simulink subsystem "Controllers"  (R2021b)
settings: Solver=VariableStepAuto  StartTime=0.0  StopTime=10.0  RelTol=1e-3
model mask{SurgeInitial=eta_IC.N, SurgeL=1.17*2, SurgeEpsilon=0.05, SurgeC0=3, SurgeAlpha=0.5, SwayInitial=eta_IC.E, SwayL=1.04, SwayEpsilon=0.03, SwayC0=3, SwayAlpha=0.5, HeaveInitial=eta_IC.D, HeaveL=0.7*5, HeaveEpsilon=0.05, HeaveC0=2, HeaveAlpha=0.1, RollInitial=eta_IC.phi, RollL=2.01, RollEpsilon=0.1, RollC0=0.4, RollAlpha=0.1, PitchInitial=eta_IC.theta, PitchL=1.83, PitchEpsilon=0.1, PitchC0=0.4, PitchAlpha=0.1, YawInitial=eta_IC.psi, YawL=2.05, YawEpsilon=0.1, YawC0=2, YawAlpha=0.1}
  mask prompts: SurgeInitial "Initial Condition"; SurgeL "L"; SurgeEpsilon "Epsilon"; SurgeC0 "C0"; SurgeAlpha "Alpha"; SwayInitial "Initial Condition"; SwayL "L"; SwayEpsilon "Epsilon"; SwayC0 "C0"; SwayAlpha "Alpha"; HeaveInitial "Initial Condition"; HeaveL "L"; HeaveEpsilon "Epsilon"; HeaveC0 "C0"; HeaveAlpha "Alpha"; RollInitial "Initial Condition"; RollL "L"; RollEpsilon "Epsilon"; RollC0 "C0"; RollAlpha "Alpha"; PitchInitial "Initial Condition"; PitchL "L"; PitchEpsilon "Epsilon"; PitchC0 "C0"; PitchAlpha "Alpha"; YawInitial "Initial Condition"; YawL "L"; YawEpsilon "Epsilon"; YawC0 "C0"; YawAlpha "Alpha"
undefined symbols (not defined in the file): eta_Init
libraries: simulink x12
settings Model: Creator=esben  LastModifiedBy=esben
settings SolverCC: AlgebraicLoopSolver=TrustRegion

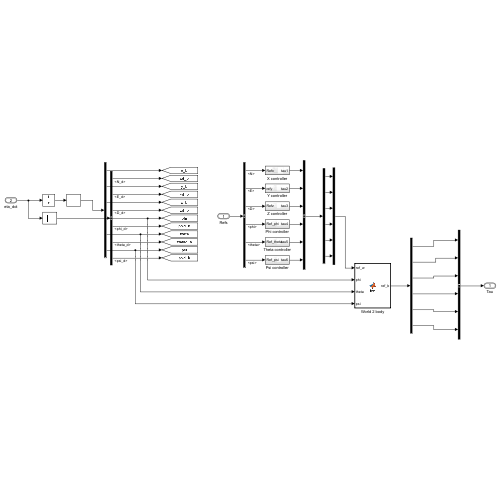
[thumbnail: Simulink's stored preview of the top-level diagram]
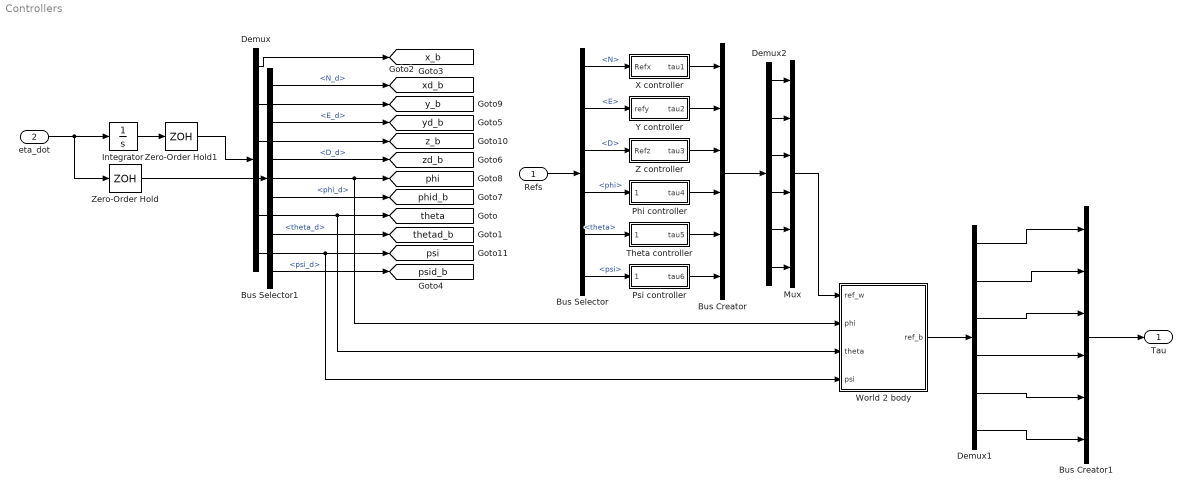
== system Controllers ==
  Refs : Inport  OutDataTypeStr=Bus: eta
  eta_dot : Inport  Port=2  OutDataTypeStr=Bus: nu
  Bus Creator : BusCreator  Inputs=6  OutDataTypeStr=Bus: tau
      settings: InheritFromInputs=off
  Bus Creator1 : BusCreator  Inputs=6  OutDataTypeStr=Bus: tau
      settings: InheritFromInputs=off
  Bus Selector : BusSelector  OutputSignals=N,E,D,phi,theta,psi
  Bus Selector1 : BusSelector  OutputSignals=N_d,E_d,D_d,phi_d,theta_d,psi_d
  Demux : Demux  Outputs=6
  Demux1 : Demux  Outputs=6
  Demux2 : Demux  Outputs=6
  Integrator : Integrator  InitialCondition=eta_Init
  Mux : Mux  Inputs=6
  Phi controller : Subsystem
  Psi controller : Subsystem
  Theta controller : Subsystem
  World 2 body : MATLAB Function  TreatAsAtomicUnit=on
  X controller : Subsystem
  Y controller : Subsystem
  Z controller : Subsystem
  Zero-Order Hold : ZeroOrderHold  SampleTime=1/20
  Zero-Order Hold1 : ZeroOrderHold  SampleTime=1/20
  Tau : Outport  OutDataTypeStr=Bus: tau
  tag scope: phi=global, phid_b=global, psi=global, psid_b=global, theta=global, thetad_b=global, x_b=global, xd_b=global, y_b=global, yd_b=global, z_b=global, zd_b=global
  wires:
  Theta controller/1(tau5) -> Bus Creator/5
  Bus Selector/5 -> Theta controller/1(Ref_theta)  "<theta>"
  Bus Selector/2 -> Y controller/1("refy ")  "<E>"
  Phi controller/1(tau4) -> Bus Creator/4
  Bus Selector/6 -> Psi controller/1(Ref_psi)  "<psi>"
  Psi controller/1(tau6) -> Bus Creator/6
  Z controller/1(tau3) -> Bus Creator/3
  Bus Selector/1 -> X controller/1(Refx)  "<N>"
  Bus Selector/4 -> Phi controller/1(Ref_phi)  "<phi>"
  Refs/1 -> Bus Selector/1
  Bus Selector/3 -> Z controller/1(Refz)  "<D>"
  eta_dot/1 -> Integrator/1, Zero-Order Hold/1
  Demux/5 -> [theta], World 2 body/3(theta)
  Bus Selector1/5 -> [thetad_b]  "<theta_d>"
  Bus Selector1/6 -> [psid_b]  "<psi_d>"
  Demux/1 -> [x_b]
  Bus Selector1/1 -> [xd_b]  "<N_d>"
  Bus Selector1/2 -> [yd_b]  "<E_d>"
  Bus Selector1/3 -> [zd_b]  "<D_d>"
  Demux/2 -> [y_b]
  Demux/3 -> [z_b]
  Demux/4 -> [phi], World 2 body/2(phi)
  Bus Selector1/4 -> [phid_b]  "<phi_d>"
  Demux/6 -> [psi], World 2 body/4(psi)
  Y controller/1(tau2) -> Bus Creator/2
  X controller/1(tau1) -> Bus Creator/1
  Zero-Order Hold/1 -> Bus Selector1/1
  Integrator/1 -> Zero-Order Hold1/1
  Zero-Order Hold1/1 -> Demux/1
  World 2 body/1(ref_b) -> Demux1/1
  Demux1/1 -> Bus Creator1/1
  Demux1/2 -> Bus Creator1/2
  Demux1/3 -> Bus Creator1/3
  Demux1/4 -> Bus Creator1/4
  Demux1/5 -> Bus Creator1/5
  Demux1/6 -> Bus Creator1/6
  Bus Creator1/1 -> Tau/1
  Bus Creator/1 -> Demux2/1
  Demux2/6 -> Mux/6
  Demux2/1 -> Mux/1
  Demux2/2 -> Mux/2
  Demux2/3 -> Mux/3
  Demux2/4 -> Mux/4
  Demux2/5 -> Mux/5
  Mux/1 -> World 2 body/1(ref_w)

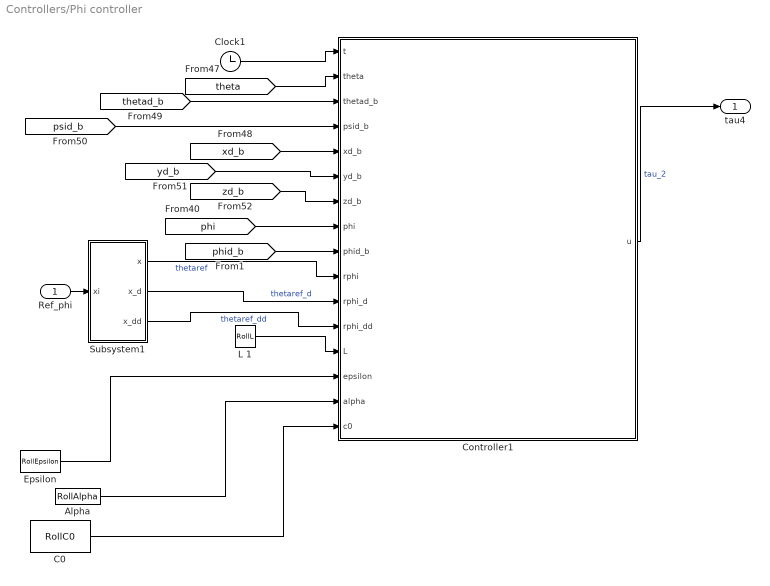
== system Controllers/Phi controller ==
  Ref_phi : Inport
  Alpha : Constant  Value=RollAlpha
  C0 : Constant  Value=RollC0
  Clock1 : Clock
  Controller1 : MATLAB Function  TreatAsAtomicUnit=on
  Epsilon : Constant  Value=RollEpsilon
  L 1 : Constant  Value=RollL
  Subsystem1 : Subsystem
  tau4 : Outport
  wires:
  C0/1 -> Controller1/16(c0)
  Epsilon/1 -> Controller1/14(epsilon)
  Alpha/1 -> Controller1/15(alpha)
  [phid_b] -> Controller1/9(phid_b)
  Controller1/1(u) -> tau4/1  "tau_2"
  Ref_phi/1 -> Subsystem1/1(xi)
  [xd_b] -> Controller1/5(xd_b)
  [psid_b] -> Controller1/4(psid_b)
  [zd_b] -> Controller1/7(zd_b)
  Subsystem1/1(x) -> Controller1/10(rphi)  "thetaref"
  [yd_b] -> Controller1/6(yd_b)
  Subsystem1/2(x_d) -> Controller1/11(rphi_d)  "thetaref_d"
  [phi] -> Controller1/8(phi)
  Clock1/1 -> Controller1/1(t)
  [thetad_b] -> Controller1/3(thetad_b)
  L 1/1 -> Controller1/13(L)
  [theta] -> Controller1/2(theta)
  Subsystem1/3(x_dd) -> Controller1/12(rphi_dd)  "thetaref_dd"

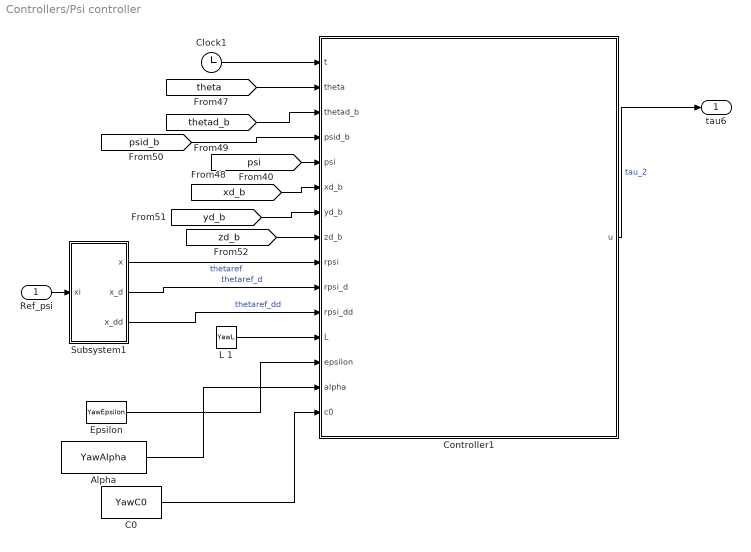
== system Controllers/Psi controller ==
  Ref_psi : Inport
  Alpha : Constant  Value=YawAlpha
  C0 : Constant  Value=YawC0
  Clock1 : Clock
  Controller1 : MATLAB Function  TreatAsAtomicUnit=on
  Epsilon : Constant  Value=YawEpsilon
  L 1 : Constant  Value=YawL
  Subsystem1 : Subsystem
  tau6 : Outport
  wires:
  Controller1/1(u) -> tau6/1  "tau_2"
  Ref_psi/1 -> Subsystem1/1(xi)
  C0/1 -> Controller1/15(c0)
  [xd_b] -> Controller1/6(xd_b)
  [psid_b] -> Controller1/4(psid_b)
  [zd_b] -> Controller1/8(zd_b)
  Subsystem1/1(x) -> Controller1/9(rpsi)  "thetaref"
  Alpha/1 -> Controller1/14(alpha)
  [yd_b] -> Controller1/7(yd_b)
  Epsilon/1 -> Controller1/13(epsilon)
  Subsystem1/2(x_d) -> Controller1/10(rpsi_d)  "thetaref_d"
  [psi] -> Controller1/5(psi)
  Clock1/1 -> Controller1/1(t)
  [thetad_b] -> Controller1/3(thetad_b)
  L 1/1 -> Controller1/12(L)
  [theta] -> Controller1/2(theta)
  Subsystem1/3(x_dd) -> Controller1/11(rpsi_dd)  "thetaref_dd"

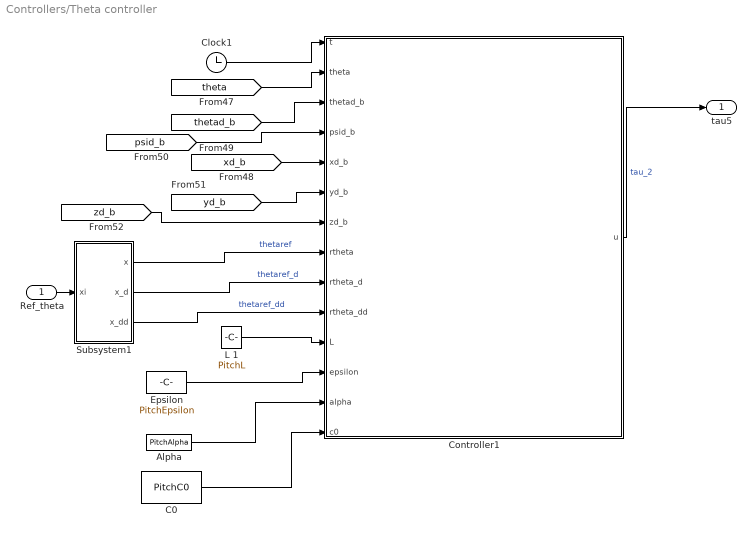
== system Controllers/Theta controller ==
  Ref_theta : Inport
  Alpha : Constant  Value=PitchAlpha
  C0 : Constant  Value=PitchC0
  Clock1 : Clock
  Controller1 : MATLAB Function  TreatAsAtomicUnit=on
  Epsilon : Constant  Value=PitchEpsilon
  L 1 : Constant  Value=PitchL
  Subsystem1 : Subsystem
  tau5 : Outport
  wires:
  C0/1 -> Controller1/14(c0)
  Epsilon/1 -> Controller1/12(epsilon)
  Alpha/1 -> Controller1/13(alpha)
  Subsystem1/2(x_d) -> Controller1/9(rtheta_d)  "thetaref_d"
  Subsystem1/3(x_dd) -> Controller1/10(rtheta_dd)  "thetaref_dd"
  [theta] -> Controller1/2(theta)
  L 1/1 -> Controller1/11(L)
  [thetad_b] -> Controller1/3(thetad_b)
  Clock1/1 -> Controller1/1(t)
  [yd_b] -> Controller1/6(yd_b)
  Subsystem1/1(x) -> Controller1/8(rtheta)  "thetaref"
  [zd_b] -> Controller1/7(zd_b)
  [psid_b] -> Controller1/4(psid_b)
  [xd_b] -> Controller1/5(xd_b)
  Ref_theta/1 -> Subsystem1/1(xi)
  Controller1/1(u) -> tau5/1  "tau_2"

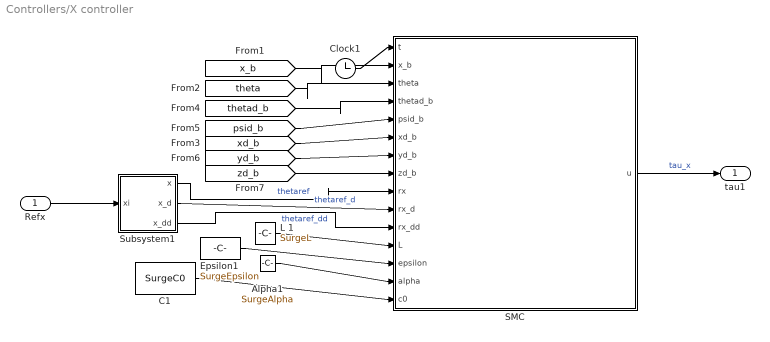
== system Controllers/X controller ==
  Refx : Inport
  Alpha1 : Constant  Value=SurgeAlpha
  C1 : Constant  Value=SurgeC0
  Clock1 : Clock
  Epsilon1 : Constant  Value=SurgeEpsilon
  L 1 : Constant  Value=SurgeL
  SMC : MATLAB Function  TreatAsAtomicUnit=on
  Subsystem1 : Subsystem
  tau1 : Outport
  wires:
  SMC/1(u) -> tau1/1  "tau_x"
  [psid_b] -> SMC/5(psid_b)
  [xd_b] -> SMC/6(xd_b)
  Epsilon1/1 -> SMC/13(epsilon)
  Clock1/1 -> SMC/1(t)
  [yd_b] -> SMC/7(yd_b)
  [thetad_b] -> SMC/4(thetad_b)
  C1/1 -> SMC/15(c0)
  L 1/1 -> SMC/12(L)
  Subsystem1/3(x_dd) -> SMC/11(rx_dd)  "thetaref_dd"
  [x_b] -> SMC/2(x_b)
  [zd_b] -> SMC/8(zd_b)
  Subsystem1/1(x) -> SMC/9(rx)  "thetaref"
  Alpha1/1 -> SMC/14(alpha)
  Subsystem1/2(x_d) -> SMC/10(rx_d)  "thetaref_d"
  Refx/1 -> Subsystem1/1(xi)
  [theta] -> SMC/3(theta)

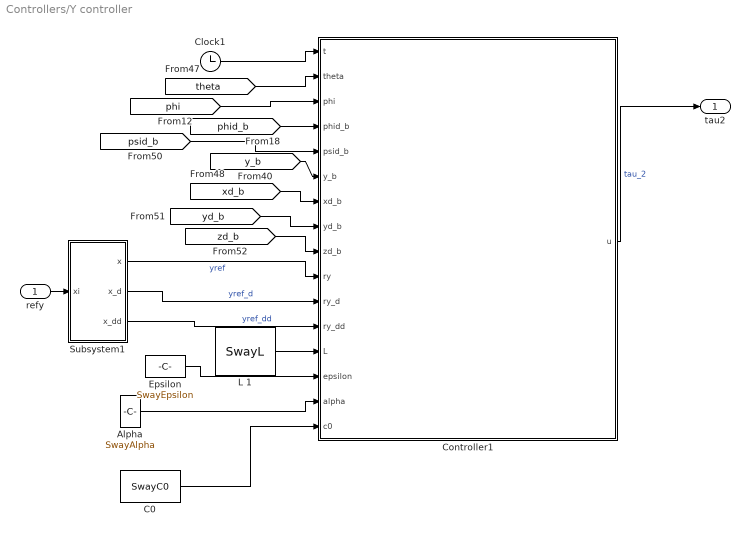
== system Controllers/Y controller ==
  "refy " : Inport
  Alpha : Constant  Value=SwayAlpha
  C0 : Constant  Value=SwayC0
  Clock1 : Clock
  Controller1 : MATLAB Function  TreatAsAtomicUnit=on
  Epsilon : Constant  Value=SwayEpsilon
  L 1 : Constant  Value=SwayL
  Subsystem1 : Subsystem
  tau2 : Outport
  wires:
  [phid_b] -> Controller1/4(phid_b)
  [phi] -> Controller1/3(phi)
  Controller1/1(u) -> tau2/1  "tau_2"
  "refy "/1 -> Subsystem1/1(xi)
  C0/1 -> Controller1/16(c0)
  [xd_b] -> Controller1/7(xd_b)
  [psid_b] -> Controller1/5(psid_b)
  [zd_b] -> Controller1/9(zd_b)
  Subsystem1/1(x) -> Controller1/10(ry)  "yref"
  Alpha/1 -> Controller1/15(alpha)
  [yd_b] -> Controller1/8(yd_b)
  Epsilon/1 -> Controller1/14(epsilon)
  Subsystem1/2(x_d) -> Controller1/11(ry_d)  "yref_d"
  [y_b] -> Controller1/6(y_b)
  Clock1/1 -> Controller1/1(t)
  L 1/1 -> Controller1/13(L)
  [theta] -> Controller1/2(theta)
  Subsystem1/3(x_dd) -> Controller1/12(ry_dd)  "yref_dd"

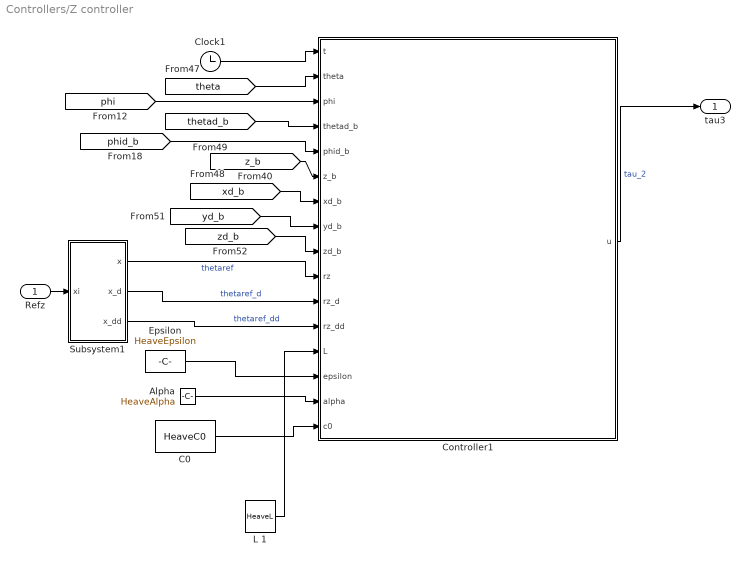
== system Controllers/Z controller ==
  Refz : Inport
  Alpha : Constant  Value=HeaveAlpha
  C0 : Constant  Value=HeaveC0
  Clock1 : Clock
  Controller1 : MATLAB Function  TreatAsAtomicUnit=on
  Epsilon : Constant  Value=HeaveEpsilon
  L 1 : Constant  Value=HeaveL
  Subsystem1 : Subsystem
  tau3 : Outport
  wires:
  [phid_b] -> Controller1/5(phid_b)
  [phi] -> Controller1/3(phi)
  Subsystem1/3(x_dd) -> Controller1/12(rz_dd)  "thetaref_dd"
  [theta] -> Controller1/2(theta)
  L 1/1 -> Controller1/13(L)
  [thetad_b] -> Controller1/4(thetad_b)
  Clock1/1 -> Controller1/1(t)
  [z_b] -> Controller1/6(z_b)
  Subsystem1/2(x_d) -> Controller1/11(rz_d)  "thetaref_d"
  Epsilon/1 -> Controller1/14(epsilon)
  [yd_b] -> Controller1/8(yd_b)
  Alpha/1 -> Controller1/15(alpha)
  Subsystem1/1(x) -> Controller1/10(rz)  "thetaref"
  [zd_b] -> Controller1/9(zd_b)
  [xd_b] -> Controller1/7(xd_b)
  C0/1 -> Controller1/16(c0)
  Refz/1 -> Subsystem1/1(xi)
  Controller1/1(u) -> tau3/1  "tau_2"

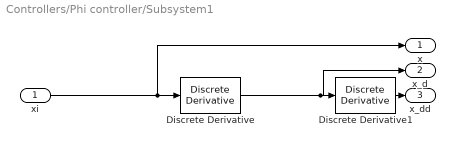
== system Controllers/Phi controller/Subsystem1 ==
  xi : Inport
  Discrete Derivative : simulink/Discrete/Discrete Derivative  gainval=1.0  ICPrevScaledInput=RollInitial  OutMin=[]  OutMax=[]  OutDataType=fixdt(1, 16)  OutScaling=2^-10  DoSatur=off
  Discrete Derivative1 : simulink/Discrete/Discrete Derivative  gainval=1.0  ICPrevScaledInput=0.0  OutMin=[]  OutMax=[]  OutDataType=fixdt(1, 16)  OutScaling=2^-10  DoSatur=off
  x : Outport
  x_d : Outport  Port=2
  x_dd : Outport  Port=3
  wires:
  xi/1 -> x/1, Discrete Derivative/1
  Discrete Derivative1/1 -> x_dd/1
  Discrete Derivative/1 -> Discrete Derivative1/1, x_d/1

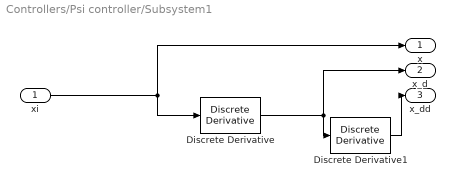
== system Controllers/Psi controller/Subsystem1 ==
  xi : Inport
  Discrete Derivative : simulink/Discrete/Discrete Derivative  gainval=1.0  ICPrevScaledInput=YawInitial  OutMin=[]  OutMax=[]  OutDataType=fixdt(1, 16)  OutScaling=2^-10  DoSatur=off
  Discrete Derivative1 : simulink/Discrete/Discrete Derivative  gainval=1.0  ICPrevScaledInput=0.0  OutMin=[]  OutMax=[]  OutDataType=fixdt(1, 16)  OutScaling=2^-10  DoSatur=off
  x : Outport
  x_d : Outport  Port=2
  x_dd : Outport  Port=3
  wires:
  xi/1 -> x/1, Discrete Derivative/1
  Discrete Derivative1/1 -> x_dd/1
  Discrete Derivative/1 -> x_d/1, Discrete Derivative1/1

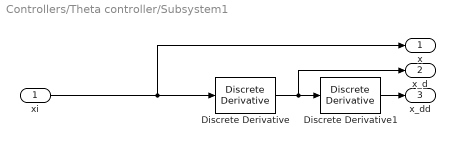
== system Controllers/Theta controller/Subsystem1 ==
  xi : Inport
  Discrete Derivative : simulink/Discrete/Discrete Derivative  gainval=1.0  ICPrevScaledInput=PitchInitial  OutMin=[]  OutMax=[]  OutDataType=fixdt(1, 16)  OutScaling=2^-10  DoSatur=off
  Discrete Derivative1 : simulink/Discrete/Discrete Derivative  gainval=1.0  ICPrevScaledInput=0.0  OutMin=[]  OutMax=[]  OutDataType=fixdt(1, 16)  OutScaling=2^-10  DoSatur=off
  x : Outport
  x_d : Outport  Port=2
  x_dd : Outport  Port=3
  wires:
  Discrete Derivative/1 -> x_d/1, Discrete Derivative1/1
  Discrete Derivative1/1 -> x_dd/1
  xi/1 -> x/1, Discrete Derivative/1

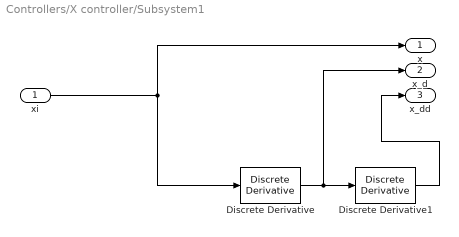
== system Controllers/X controller/Subsystem1 ==
  xi : Inport
  Discrete Derivative : simulink/Discrete/Discrete Derivative  gainval=1.0  ICPrevScaledInput=SurgeInitial  OutMin=[]  OutMax=[]  OutDataType=fixdt(1, 16)  OutScaling=2^-10  DoSatur=off
  Discrete Derivative1 : simulink/Discrete/Discrete Derivative  gainval=1.0  ICPrevScaledInput=0.0  OutMin=[]  OutMax=[]  OutDataType=fixdt(1, 16)  OutScaling=2^-10  DoSatur=off
  x : Outport
  x_d : Outport  Port=2
  x_dd : Outport  Port=3
  wires:
  xi/1 -> x/1, Discrete Derivative/1
  Discrete Derivative1/1 -> x_dd/1
  Discrete Derivative/1 -> Discrete Derivative1/1, x_d/1

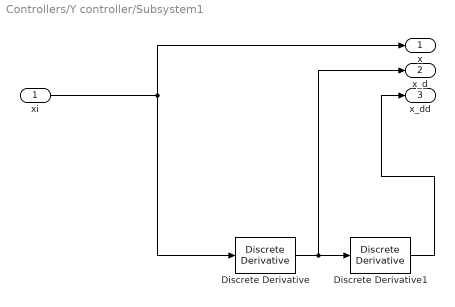
== system Controllers/Y controller/Subsystem1 ==
  xi : Inport
  Discrete Derivative : simulink/Discrete/Discrete Derivative  gainval=1.0  ICPrevScaledInput=SwayInitial  OutMin=[]  OutMax=[]  OutDataType=fixdt(1, 16)  OutScaling=2^-10  DoSatur=off
  Discrete Derivative1 : simulink/Discrete/Discrete Derivative  gainval=1.0  ICPrevScaledInput=0.0  OutMin=[]  OutMax=[]  OutDataType=fixdt(1, 16)  OutScaling=2^-10  DoSatur=off
  x : Outport
  x_d : Outport  Port=2
  x_dd : Outport  Port=3
  wires:
  Discrete Derivative1/1 -> x_dd/1
  Discrete Derivative/1 -> Discrete Derivative1/1, x_d/1
  xi/1 -> Discrete Derivative/1, x/1

== system Controllers/Z controller/Subsystem1 ==
  xi : Inport
  Discrete Derivative : simulink/Discrete/Discrete Derivative  gainval=1.0  ICPrevScaledInput=HeaveInitial  OutMin=[]  OutMax=[]  OutDataType=fixdt(1, 16)  OutScaling=2^-10  DoSatur=off
  Discrete Derivative1 : simulink/Discrete/Discrete Derivative  gainval=1.0  ICPrevScaledInput=0.0  OutMin=[]  OutMax=[]  OutDataType=fixdt(1, 16)  OutScaling=2^-10  DoSatur=off
  x : Outport
  x_d : Outport  Port=2
  x_dd : Outport  Port=3
  wires:
  Discrete Derivative1/1 -> x_dd/1
  Discrete Derivative/1 -> Discrete Derivative1/1, x_d/1
  xi/1 -> x/1, Discrete Derivative/1

== matlab function Controllers/Phi controller/Controller1 ==
  data: t input; theta input; thetad_b input; psid_b input; xd_b input; yd_b input; zd_b input; phi input; phid_b input; rphi input; rphi_d input; rphi_dd input; u output; L input; epsilon input; alpha input; c0 input
function u = fcn(t,theta,thetad_b,psid_b,xd_b,yd_b,zd_b,phi,phid_b,rphi,rphi_d,rphi_dd,L,epsilon,alpha,c0)
%#codegen   

% ASMC
f = -0.064291*sin(theta) - 0.050361*xd_b*(32.78*abs(xd_b) + 26.1) + 1.6209*psid_b*yd_b - 1.0385*thetad_b*zd_b;
gt =2.2433;
% Control error(s)
e = phi-rphi;
e_d = phid_b-rphi_d;

% Original constraint function(s)
sigma = e_d+c0*e;
%Se slide 8+9 Lek 13 (vi antager at g(t)=g_hat(t), derfor alpha_m = r_dd-c0*e-d+v
%sigma_d = f+v;

% Sliding constraint
%S = sigma_d+k0*sigma;

% sgn-function
%sgn = (S>=0)-(S<0);
% Switching gain
rho = alpha/sqrt(2)+L;

v = -rho*(sigma)/(abs(sigma)+epsilon);%-rho*sgn(sigma)%

% Control input signal
u = gt^-1*(rphi_dd-c0*e_d+v);

== matlab function Controllers/Theta controller/Controller1 ==
  data: t input; theta input; thetad_b input; psid_b input; xd_b input; yd_b input; zd_b input; rtheta input; rtheta_d input; rtheta_dd input; u output; L input; epsilon input; alpha input; c0 input
function u = fcn(t,theta,thetad_b,psid_b,xd_b,yd_b,zd_b,rtheta,rtheta_d,rtheta_dd,L,epsilon,alpha,c0)
%#codegen   

% ASMC
f = -0.064291*sin(theta) - 0.050361*xd_b*(32.78*abs(xd_b) + 26.1) + 1.6209*psid_b*yd_b - 1.0385*thetad_b*zd_b;
gt= 2.7410526;
% Control error(s)
e = theta-rtheta;
e_d = thetad_b-rtheta_d;

% Original constraint function(s)
sigma = e_d+c0*e;
%Se slide 8+9 Lek 13 (vi antager at g(t)=g_hat(t), derfor alpha_m = r_dd-c0*e-d+v
%sigma_d = f+v;

% Sliding constraint
%S = sigma_d+k0*sigma;

% sgn-function
%sgn = (S>=0)-(S<0);
% Switching gain
rho = alpha/sqrt(2)+L;

v = -rho*(sigma)/(abs(sigma)+epsilon);%-rho*sgn(sigma)%

% Control input signal
u = gt^-1*(rtheta_dd-c0*e_d+v);

== matlab function Controllers/Psi controller/Controller1 ==
  data: t input; theta input; thetad_b input; psid_b input; psi input; xd_b input; yd_b input; zd_b input; rpsi input; rpsi_d input; rpsi_dd input; u output; L input; epsilon input; alpha input; c0 input
function u = fcn(t,theta,thetad_b,psid_b,psi,xd_b,yd_b,zd_b,rpsi,rpsi_d,rpsi_dd,L,epsilon,alpha,c0)
%#codegen   

% ASMC
f = -0.064291*sin(theta) - 0.050361*xd_b*(32.78*abs(xd_b) + 26.1) + 1.6209*psid_b*yd_b - 1.0385*thetad_b*zd_b;
gt =1.690587;
% Control error(s)
e = psi-rpsi;
e_d = psid_b-rpsi_d;

% Original constraint function(s)
sigma = e_d+c0*e;
%Se slide 8+9 Lek 13 (vi antager at g(t)=g_hat(t), derfor alpha_m = r_dd-c0*e-d+v
%sigma_d = f+v;

% Sliding constraint
%S = sigma_d+k0*sigma;

% sgn-function
%sgn = (S>=0)-(S<0);
% Switching gain
rho = alpha/sqrt(2)+L;

v = -rho*(sigma)/(abs(sigma)+epsilon);%-rho*sgn(sigma)%

% Control input signal
u = gt^-1*(rpsi_dd-c0*e_d+v);

== matlab function Controllers/World 2 body ==
  data: ref_w input; ref_b output; phi input; theta input; psi input
function ref_b = fcn(ref_w, phi,theta,psi)

J_Tinv=[                              cos(psi)*cos(theta)                              cos(theta)*sin(psi)         -sin(theta) 0         0                  0;
 cos(psi)*sin(phi)*sin(theta) - cos(phi)*sin(psi) cos(phi)*cos(psi) + sin(phi)*sin(psi)*sin(theta) cos(theta)*sin(phi) 0         0                  0;
 sin(phi)*sin(psi) + cos(phi)*cos(psi)*sin(theta) cos(phi)*sin(psi)*sin(theta) - cos(psi)*sin(phi) cos(phi)*cos(theta) 0         0                   0;
                                                0                                                0                   0 1         0         -sin(theta);
                                                0                                                0                   0 0  cos(phi) cos(theta)*sin(phi);
                                                0                                                0                   0 0 -sin(phi) cos(phi)*cos(theta)];


ref_b=J_Tinv*ref_w;

== matlab function Controllers/Y controller/Controller1 ==
  data: t input; theta input; phi input; phid_b input; psid_b input; y_b input; xd_b input; yd_b input; zd_b input; ry input; ry_d input; ry_dd input; u output; L input; epsilon input; alpha input; c0 input
function u = fcn(t,theta,phi,phid_b,psid_b,y_b,xd_b,yd_b,zd_b,ry,ry_d,ry_dd,L,epsilon,alpha,c0)
%#codegen   

% ASMC
f = 0.061908963933639427068555960431695*cos(theta)*sin(phi) - 0.048495193430703409376292256638408*yd_b*(50.940000000002328306436538696289*abs(yd_b) + 20.0) - 1.5608821469741087639704346656799*psid_b*xd_b + 0.96295324102777613006765022873878*phid_b*zd_b;
gt =0.048495193430703409376292256638408;
% Control error(s)
e = y_b-ry;
e_d = yd_b-ry_d;

% Original constraint function(s)
sigma = e_d+c0*e;
%Se slide 8+9 Lek 13 (vi antager at g(t)=g_hat(t), derfor alpha_m = r_dd-c0*e-d+v
%sigma_d = f+v;

% Sliding constraint
%S = sigma_d+k0*sigma;

% sgn-function
%sgn = (S>=0)-(S<0);
% Switching gain
rho = alpha/sqrt(2)+L;

v = -rho*(sigma)/(abs(sigma)+epsilon);%-rho*sgn(sigma)%

% Control input signal
u = gt^-1*(ry_dd-c0*e_d+v);

== matlab function Controllers/Z controller/Controller1 ==
  data: t input; theta input; phi input; thetad_b input; phid_b input; z_b input; xd_b input; yd_b input; zd_b input; rz input; rz_d input; rz_dd input; u output; L input; epsilon input; alpha input; c0 input
function u = fcn(t,theta,phi,thetad_b,phid_b,z_b,xd_b,yd_b,zd_b,rz,rz_d,rz_dd,L,epsilon,alpha,c0)
%#codegen   

% ASMC
f = 0.039662804814355467897257767617702*cos(phi)*cos(theta) - 0.031069093540931902452939539216459*zd_b*(47.330000000001746229827404022217*abs(zd_b) + 36.339999999996507540345191955566) - 0.61692885839886457688407972455025*phid_b*yd_b + 0.64066335945904029358644038438797*thetad_b*xd_b;
gt =0.031069093540931902452939539216459;
% Control error(s)
e = z_b-rz;
e_d = zd_b-rz_d;

% Original constraint function(s)
sigma = e_d+c0*e;
%Se slide 8+9 Lek 13 (vi antager at g(t)=g_hat(t), derfor alpha_m = r_dd-c0*e-d+v
%sigma_d = f+v;

% Sliding constraint
%S = sigma_d+k0*sigma;

% sgn-function
%sgn = (S>=0)-(S<0);
% Switching gain
rho = alpha/sqrt(2)+L;

v = -rho*(sigma)/(abs(sigma)+epsilon);%-rho*sgn(sigma)%

% Control input signal
u = gt^-1*(rz_dd-c0*e_d+v);

== matlab function Controllers/X controller/SMC ==
  data: t input; x_b input; theta input; thetad_b input; psid_b input; xd_b input; yd_b input; zd_b input; rx input; rx_d input; rx_dd input; u output; L input; epsilon input; alpha input; c0 input
function u = fcn(t,x_b,theta,thetad_b,psid_b,xd_b,yd_b,zd_b,rx,rx_d,rx_dd,L,epsilon,alpha,c0)
%#codegen   

% ASMC
f = 1.6209324404039762157481163740158*psid_b*yd_b - 0.050360901614439512741228099912405*xd_b*(32.779999999998835846781730651855*abs(xd_b) + 26.099999999998544808477163314819) - 0.064290727000994252193777356296778*sin(theta) - 1.0384720227252728363964706659317*thetad_b*zd_b;
gt =0.050360901614439512741228099912405*1;
% Control error(s)
e = x_b-rx;
e_d = xd_b-rx_d;

% Original constraint function(s)
sigma = e_d+c0*e;
%Se slide 8+9 Lek 13 (vi antager at g(t)=g_hat(t), derfor alpha_m = r_dd-c0*e-d+v
%sigma_d = f+v;

% Sliding constraint
%S = sigma_d+k0*sigma;

% sgn-function
%sgn = (S>=0)-(S<0);
% Switching gain
rho = alpha/sqrt(2)+L;

v = -rho*(sigma)/(abs(sigma)+epsilon);%-rho*sgn(sigma)%

% Control input signal
u = gt^-1*(rx_dd-c0*e_d+v);
